simulink model "mandelbrot"  (R2020a)
settings: Solver=VariableStepAuto  StartTime=0.0  StopTime=500.0  RelTol=1e-3
undefined symbols (not defined in the file): AXI4, Lite
libraries: xbsIndex_r4 x38
settings Model: Creator=cwb21157  LastModifiedBy=cwb21157

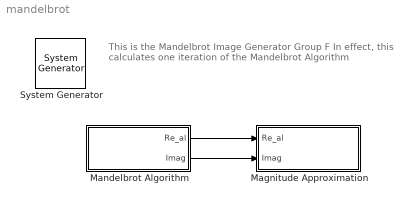
== system mandelbrot ==
  note: This is the Mandelbrot Image Generator
      | Group F
      |
      | In effect, this calculates one iteration of the Mandelbrot Algorithm
  " System Generator" : xbsIndex_r4/ System Generator  Tag=genX  xilinxfamily=zynq  part=xc7z020  speed=-1  package=clg400  synthesis_tool=Vivado  clock_wrapper=Clock Enables  directory=C:/Users/cwb21157/MANDELPROJECT/MandelBrotFinal  proj_type=Vivado  Synth_file=Vivado Synthesis Defaults  Impl_file=Vivado Implementation Defaults  testbench=off  simulink_period=1  sysclk_period=10  dcm_input_clock_period=10  incr_netlist=off  trim_vbits=Everywhere in SubSystem  dbl_ovrd=According to Block Masks  core_generation=According to Block Masks  run_coregen=off  deprecated_control=off  eval_field=0  block_type=sysgen
  Magnitude Approximation : Subsystem
  Mandelbrot Algorithm : Subsystem
  wires:
  Mandelbrot Algorithm/1(Re_al) -> Magnitude Approximation/1(Re_al)
  Mandelbrot Algorithm/2(Imag) -> Magnitude Approximation/2(Imag)

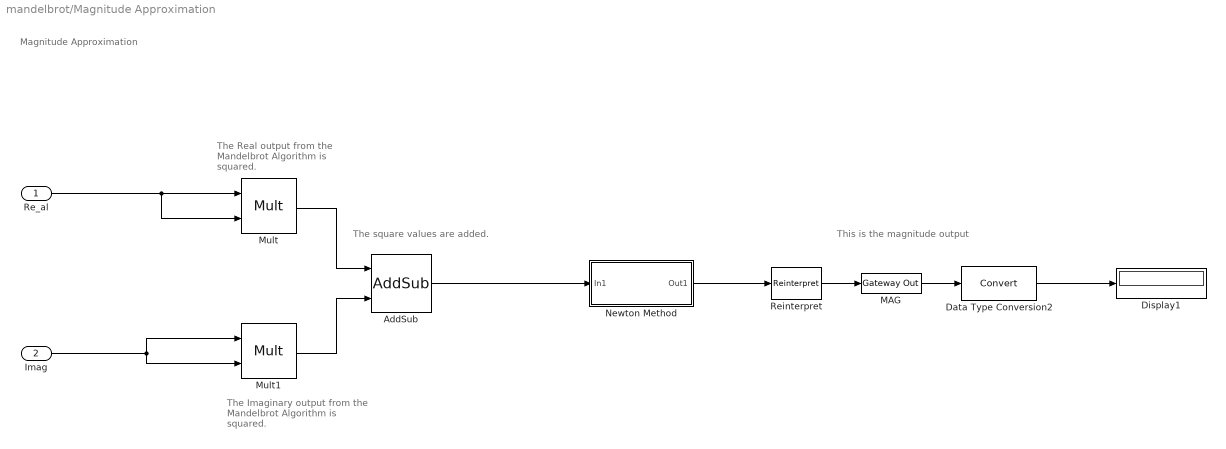
== system mandelbrot/Magnitude Approximation ==
  note: This is the magnitude output
  note: The square values are added.
  note: The Imaginary output from the Mandelbrot Algorithm is squared.
  note: The Real output from the Mandelbrot Algorithm is squared.
  note: Magnitude Approximation
  Re_al : Inport
  Imag : Inport  Port=2
  AddSub : xbsIndex_r4/AddSub  mode=Addition  use_carryin=off  use_carryout=off  en=off  latency=1  precision=Full  arith_type=Unsigned  n_bits=16  bin_pt=14  quantization=Truncate  overflow=Wrap  use_behavioral_HDL=off  hw_selection=DSP48  pipelined=off  dbl_ovrd=off  block_type=addsub
  Data Type Conversion2 : DataTypeConversion  ConvertRealWorld=Stored Integer (SI)
  Display1 : Display
  MAG : xbsIndex_r4/Gateway Out  inherit_from_input=off  hdl_port=on  rows=1  columns=1  UseAsDAC=off  DACChannel='1'  interface=AXI4-Lite  automatic_assignment=on  address_offset=hex2dec('00')  intf_name=''  intf_description=''  timing_constraint=None  locs_specified=off  LOCs={}  io_standard={}  block_type=gatewayout
  Mult : xbsIndex_r4/Mult  precision=User Defined  arith_type=Unsigned  n_bits=32  bin_pt=9  quantization=Truncate  overflow=Wrap  en=off  latency=3  use_behavioral_HDL=off  opt=Speed  use_embedded=on  optimum_pipeline=off  pipeline=on  dbl_ovrd=off  use_rpm=on  placement_style=Triangular  block_type=mult
  Mult1 : xbsIndex_r4/Mult  precision=User Defined  arith_type=Unsigned  n_bits=32  bin_pt=9  quantization=Truncate  overflow=Wrap  en=off  latency=3  use_behavioral_HDL=off  opt=Speed  use_embedded=on  optimum_pipeline=off  pipeline=on  dbl_ovrd=off  use_rpm=on  placement_style=Triangular  block_type=mult
  Newton Method : Subsystem
  Reinterpret : xbsIndex_r4/Reinterpret  force_arith_type=on  arith_type=Unsigned  force_bin_pt=on  bin_pt=0  block_type=reinterpret
  wires:
  Imag/1 -> Mult1/2, Mult1/1
  Re_al/1 -> Mult/2, Mult/1
  Mult/1 -> AddSub/1
  Mult1/1 -> AddSub/2
  Data Type Conversion2/1 -> Display1/1
  Reinterpret/1 -> MAG/1
  MAG/1 -> Data Type Conversion2/1
  AddSub/1 -> Newton Method/1(In1)
  Newton Method/1(Out1) -> Reinterpret/1

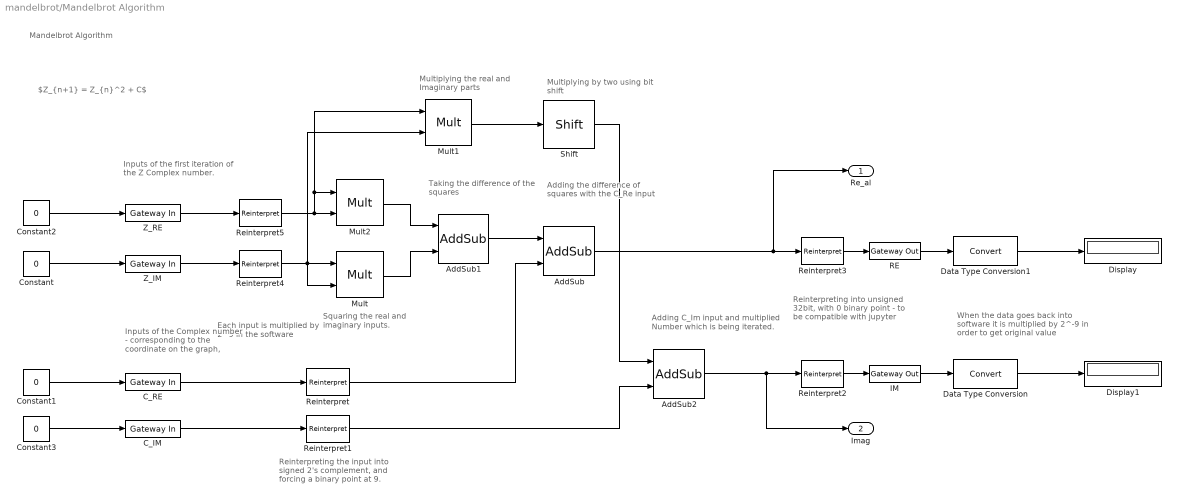
== system mandelbrot/Mandelbrot Algorithm ==
  note: $Z_{n+1} = Z_{n}^2 + C$
  note: When the data goes back into software it is multiplied by 2^-9 in order to get original value
  note: Each input is multiplied by 2^9 in the software
  note: Reinterpreting into unsigned 32bit, with 0 binary point - to be compatible with jupyter
  note: Adding C_Im input and multiplied Number which is being iterated.
  note: Adding the difference of squares with the C_Re input
  note: Taking the difference of the squares
  note: Multiplying by two using bit shift
  note: Multiplying the real and Imaginary parts
  note: Squaring the real and imaginary inputs.
  note: Reinterpreting the input into signed 2's complement, and forcing a binary point at 9.
  note: Inputs of the Complex number - corresponding to the coordinate on the graph,
  note: Inputs of the first iteration of the Z Complex number.
  note: Mandelbrot Algorithm
  AddSub : xbsIndex_r4/AddSub  mode=Addition  use_carryin=off  use_carryout=off  en=off  latency=1  precision=User Defined  arith_type="Signed  (2's comp)"  n_bits=32  bin_pt=9  quantization=Truncate  overflow=Wrap  use_behavioral_HDL=off  hw_selection=DSP48  pipelined=off  dbl_ovrd=off  block_type=addsub
  AddSub1 : xbsIndex_r4/AddSub  mode=Subtraction  use_carryin=off  use_carryout=off  en=off  latency=1  precision=User Defined  arith_type="Signed  (2's comp)"  n_bits=32  bin_pt=9  quantization=Truncate  overflow=Wrap  use_behavioral_HDL=off  hw_selection=DSP48  pipelined=off  dbl_ovrd=off  block_type=addsub
  AddSub2 : xbsIndex_r4/AddSub  mode=Addition  use_carryin=off  use_carryout=off  en=off  latency=1  precision=User Defined  arith_type="Signed  (2's comp)"  n_bits=32  bin_pt=9  quantization=Truncate  overflow=Wrap  use_behavioral_HDL=off  hw_selection=DSP48  pipelined=off  dbl_ovrd=off  block_type=addsub
  C_IM : xbsIndex_r4/Gateway In  gui_display_data_type=Fixed-point  arith_type="Signed  (2's comp)"  n_bits=32  bin_pt=0  preci_type=Single  exp_width=8  frac_width=24  rows=1  columns=1  quantization="Round  (unbiased: +/- Inf)"  overflow=Saturate  period=1  UseAsADC=off  ADCChannel='1'  interface=AXI4-Lite  automatic_assignment=on  address_offset=hex2dec('00')  intf_name=''  intf_description=''  default_value=0  timing_constraint=None  locs_specified=off  LOCs={}  io_standard={}  inherit_from_input=off  hdl_port=on  dbl_ovrd=off  block_type=gatewayin
  C_RE : xbsIndex_r4/Gateway In  gui_display_data_type=Fixed-point  arith_type="Signed  (2's comp)"  n_bits=32  bin_pt=0  preci_type=Single  exp_width=8  frac_width=24  rows=1  columns=1  quantization="Round  (unbiased: +/- Inf)"  overflow=Saturate  period=1  UseAsADC=off  ADCChannel='1'  interface=AXI4-Lite  automatic_assignment=on  address_offset=hex2dec('00')  intf_name=''  intf_description=''  default_value=0  timing_constraint=None  locs_specified=off  LOCs={}  io_standard={}  inherit_from_input=off  hdl_port=on  dbl_ovrd=off  block_type=gatewayin
  Constant{,1..3} (4 alike) : Constant  Value=0
  Data Type Conversion : DataTypeConversion  ConvertRealWorld=Stored Integer (SI)
  Data Type Conversion1 : DataTypeConversion  ConvertRealWorld=Stored Integer (SI)
  Display : Display
  Display1 : Display
  IM : xbsIndex_r4/Gateway Out  inherit_from_input=off  hdl_port=on  rows=1  columns=1  UseAsDAC=off  DACChannel='1'  interface=AXI4-Lite  automatic_assignment=on  address_offset=hex2dec('00')  intf_name=''  intf_description=''  timing_constraint=None  locs_specified=off  LOCs={}  io_standard={}  block_type=gatewayout
  Mult : xbsIndex_r4/Mult  precision=User Defined  arith_type="Signed  (2's comp)"  n_bits=32  bin_pt=9  quantization=Truncate  overflow=Wrap  en=off  latency=3  use_behavioral_HDL=off  opt=Speed  use_embedded=on  optimum_pipeline=off  pipeline=on  dbl_ovrd=off  use_rpm=on  placement_style=Triangular  block_type=mult
  Mult1 : xbsIndex_r4/Mult  precision=User Defined  arith_type="Signed  (2's comp)"  n_bits=32  bin_pt=9  quantization=Truncate  overflow=Wrap  en=off  latency=3  use_behavioral_HDL=off  opt=Speed  use_embedded=on  optimum_pipeline=off  pipeline=on  dbl_ovrd=off  use_rpm=on  placement_style=Triangular  block_type=mult
  Mult2 : xbsIndex_r4/Mult  precision=User Defined  arith_type="Signed  (2's comp)"  n_bits=32  bin_pt=9  quantization=Truncate  overflow=Wrap  en=off  latency=3  use_behavioral_HDL=off  opt=Speed  use_embedded=on  optimum_pipeline=off  pipeline=on  dbl_ovrd=off  use_rpm=on  placement_style=Triangular  block_type=mult
  RE : xbsIndex_r4/Gateway Out  inherit_from_input=off  hdl_port=on  rows=1  columns=1  UseAsDAC=off  DACChannel='1'  interface=AXI4-Lite  automatic_assignment=on  address_offset=hex2dec('00')  intf_name=''  intf_description=''  timing_constraint=None  locs_specified=off  LOCs={}  io_standard={}  block_type=gatewayout
  Reinterpret{,1,4..5} (4 alike) : xbsIndex_r4/Reinterpret  force_arith_type=on  arith_type="Signed  (2's comp)"  force_bin_pt=on  bin_pt=9  block_type=reinterpret
  Reinterpret2 : xbsIndex_r4/Reinterpret  force_arith_type=on  arith_type=Unsigned  force_bin_pt=on  bin_pt=0  block_type=reinterpret
  Reinterpret3 : xbsIndex_r4/Reinterpret  force_arith_type=on  arith_type=Unsigned  force_bin_pt=on  bin_pt=0  block_type=reinterpret
  Shift : xbsIndex_r4/Shift  shift_dir=Left  shift_bits=1  en=off  latency=1  precision=User Defined  arith_type="Signed  (2's comp)"  n_bits=32  bin_pt=9  quantization=Truncate  overflow=Wrap  dbl_ovrd=off  block_type=shift
  Z_IM : xbsIndex_r4/Gateway In  gui_display_data_type=Fixed-point  arith_type="Signed  (2's comp)"  n_bits=32  bin_pt=0  preci_type=Single  exp_width=8  frac_width=24  rows=1  columns=1  quantization="Round  (unbiased: +/- Inf)"  overflow=Saturate  period=1  UseAsADC=off  ADCChannel='1'  interface=AXI4-Lite  automatic_assignment=on  address_offset=hex2dec('00')  intf_name=''  intf_description=''  default_value=0  timing_constraint=None  locs_specified=off  LOCs={}  io_standard={}  inherit_from_input=off  hdl_port=on  dbl_ovrd=off  block_type=gatewayin
  Z_RE : xbsIndex_r4/Gateway In  gui_display_data_type=Fixed-point  arith_type="Signed  (2's comp)"  n_bits=32  bin_pt=0  preci_type=Single  exp_width=8  frac_width=24  rows=1  columns=1  quantization="Round  (unbiased: +/- Inf)"  overflow=Saturate  period=1  UseAsADC=off  ADCChannel='1'  interface=AXI4-Lite  automatic_assignment=on  address_offset=hex2dec('00')  intf_name=''  intf_description=''  default_value=0  timing_constraint=None  locs_specified=off  LOCs={}  io_standard={}  inherit_from_input=off  hdl_port=on  dbl_ovrd=off  block_type=gatewayin
  Re_al : Outport
  Imag : Outport  Port=2
  wires:
  Z_RE/1 -> Reinterpret5/1
  Z_IM/1 -> Reinterpret4/1
  Mult1/1 -> Shift/1
  Mult2/1 -> AddSub1/1
  Mult/1 -> AddSub1/2
  AddSub1/1 -> AddSub/1
  Constant1/1 -> C_RE/1
  Constant3/1 -> C_IM/1
  C_RE/1 -> Reinterpret/1
  C_IM/1 -> Reinterpret1/1
  Shift/1 -> AddSub2/1
  AddSub2/1 -> Reinterpret2/1, Imag/1
  AddSub/1 -> Reinterpret3/1, Re_al/1
  IM/1 -> Data Type Conversion/1
  RE/1 -> Data Type Conversion1/1
  Data Type Conversion1/1 -> Display/1
  Data Type Conversion/1 -> Display1/1
  Reinterpret5/1 -> Mult1/1, Mult2/1, Mult2/2
  Reinterpret4/1 -> Mult/2, Mult1/2, Mult/1
  Reinterpret/1 -> AddSub/2
  Reinterpret1/1 -> AddSub2/2
  Reinterpret3/1 -> RE/1
  Constant2/1 -> Z_RE/1
  Constant/1 -> Z_IM/1
  Reinterpret2/1 -> IM/1

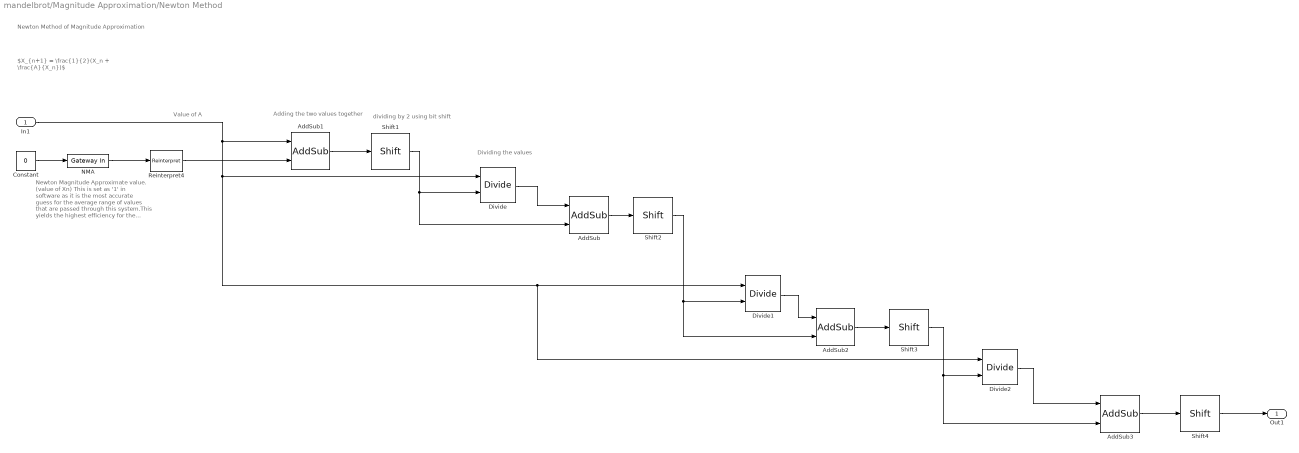
== system mandelbrot/Magnitude Approximation/Newton Method ==
  note: Dividing the values
  note: Adding the two values together
  note: dividing by 2 using bit shift
  note: Value of A
  note: $X_{n+1} = \frac{1}{2}(X_n + \frac{A}{X_n})$
  note: Newton Magnitude Approximate value. (value of Xn)
      | This is set as '1' in software as it is the most accurate guess for the average range of values that are passed through this system.This yields the highest efficiency for the algorithm utilisng the minimum amount of resources.
  note: Newton Method of Magnitude Approximation
  In1 : Inport
  AddSub{,1..3} (4 alike) : xbsIndex_r4/AddSub  mode=Addition  use_carryin=off  use_carryout=off  en=off  latency=1  precision=User Defined  arith_type=Unsigned  n_bits=32  bin_pt=9  quantization=Truncate  overflow=Wrap  use_behavioral_HDL=off  hw_selection=Fabric  pipelined=off  dbl_ovrd=off  block_type=addsub
  Constant : Constant  Value=0
  Divide : xbsIndex_r4/Divide  flow_control=NonBlocking  axi_optimize_goal=Resources  algorithm_type=Radix2  infoedit1=Specify output fraction-width for Fixed-point division.  fractional_width=16  infoedit2=Specify latency for Floating-point division.  latency=1  rate=1  has_a_tlast=off  has_a_tuser=off  has_b_tlast=off  has_b_tuser=off  en=off  has_result_tready=off  result_tlast_behv=Pass_A_TLAST  has_underflow=off  has_overflow=off  has_invalid_op=off  has_divide_by_zero=off  fpo_op_type=mergeddivide  block_type=divide
      settings: infoedit=Blocking: Wait for data on all inputs, allow back-pressure.<br>NonBlocking: operate every cycle in which all inputs are valid, no back-pressure.
  Divide1 : xbsIndex_r4/Divide  flow_control=NonBlocking  axi_optimize_goal=Resources  algorithm_type=Radix2  infoedit1=Specify output fraction-width for Fixed-point division.  fractional_width=16  infoedit2=Specify latency for Floating-point division.  latency=1  rate=1  has_a_tlast=off  has_a_tuser=off  has_b_tlast=off  has_b_tuser=off  en=off  has_result_tready=off  result_tlast_behv=Pass_A_TLAST  has_underflow=off  has_overflow=off  has_invalid_op=off  has_divide_by_zero=off  fpo_op_type=mergeddivide  block_type=divide
      settings: infoedit=Blocking: Wait for data on all inputs, allow back-pressure.<br>NonBlocking: operate every cycle in which all inputs are valid, no back-pressure.
  Divide2 : xbsIndex_r4/Divide  flow_control=NonBlocking  axi_optimize_goal=Resources  algorithm_type=Radix2  infoedit1=Specify output fraction-width for Fixed-point division.  fractional_width=16  infoedit2=Specify latency for Floating-point division.  latency=1  rate=1  has_a_tlast=off  has_a_tuser=off  has_b_tlast=off  has_b_tuser=off  en=off  has_result_tready=off  result_tlast_behv=Pass_A_TLAST  has_underflow=off  has_overflow=off  has_invalid_op=off  has_divide_by_zero=off  fpo_op_type=mergeddivide  block_type=divide
      settings: infoedit=Blocking: Wait for data on all inputs, allow back-pressure.<br>NonBlocking: operate every cycle in which all inputs are valid, no back-pressure.
  NMA : xbsIndex_r4/Gateway In  gui_display_data_type=Fixed-point  arith_type=Unsigned  n_bits=32  bin_pt=0  preci_type=Single  exp_width=8  frac_width=24  rows=1  columns=1  quantization="Round  (unbiased: +/- Inf)"  overflow=Saturate  period=1  UseAsADC=off  ADCChannel='1'  interface=AXI4-Lite  automatic_assignment=on  address_offset=hex2dec('00')  intf_name=''  intf_description=''  default_value=0  timing_constraint=None  locs_specified=off  LOCs={}  io_standard={}  inherit_from_input=off  hdl_port=on  dbl_ovrd=off  block_type=gatewayin
  Reinterpret4 : xbsIndex_r4/Reinterpret  force_arith_type=on  arith_type=Unsigned  force_bin_pt=on  bin_pt=9  block_type=reinterpret
  Shift{1..4} (4 alike) : xbsIndex_r4/Shift  shift_dir=Left  shift_bits=-1  en=off  latency=1  precision=User Defined  arith_type=Unsigned  n_bits=32  bin_pt=9  quantization=Truncate  overflow=Wrap  dbl_ovrd=off  block_type=shift
  Out1 : Outport
  wires:
  Constant/1 -> NMA/1
  In1/1 -> AddSub1/1, Divide2/1, Divide1/1, Divide/1
  AddSub1/1 -> Shift1/1
  Shift1/1 -> AddSub/2, Divide/2
  Divide/1 -> AddSub/1
  AddSub/1 -> Shift2/1
  Divide1/1 -> AddSub2/1
  AddSub2/1 -> Shift3/1
  AddSub3/1 -> Shift4/1
  Divide2/1 -> AddSub3/1
  Shift4/1 -> Out1/1
  NMA/1 -> Reinterpret4/1
  Reinterpret4/1 -> AddSub1/2
  Shift2/1 -> AddSub2/2, Divide1/2
  Shift3/1 -> AddSub3/2, Divide2/2
